simulink model "ct_finite_horizon"  (Simulink 8.7)
settings: Solver=ode45  StartTime=0.0  StopTime=5  MaxStep=1e-3  RelTol=1e-3
values from neighbouring files (symbols this model uses):
  p12 = fliplr(p12_acc)    [LUT_hint.m]    (also in Riccati_sol2.m)
  p22 = fliplr(p22_acc)    [LUT_hint.m]    (also in Riccati_sol2.m)
  Q = [2 1; 1 4]    [Riccati_sol2.m]    (also in file_for_LQR_EX.m = [100 0 ; 0 0]; inf_horiz.m = [10 0; 0 2000])
  R = 1/2    (= 0.5)    [Riccati_sol2.m]    (also in file_for_LQR_EX.m = 10; inf_horiz.m = 1)
  tt = fliplr(t_acc)    [LUT_hint.m]    (also in Riccati_sol2.m)
  Z = [p11_old p12_old; p12_old, p22_old]    [Riccati_sol2.m]
settings Model: Creator=Thomas Chmielewski  LastModifiedBy=DR_C
settings DataIOCC: SignalLoggingSaveFormat=ModelDataLogs  SignalLoggingName=sigsOut
settings OptimizationCC: ExpressionDepthLimit=2147483647  InitFltsAndDblsToZero=on
settings DebuggingCC: SaveWithParameterizedLinksMsg=none  SignalResolutionControl=TryResolveAllWithWarning  MultiTaskDSMMsg=warning  MultiTaskCondExecSysMsg=none  FcnCallInpInsideContextMsg=UseLocalSettings  StateNameClashWarn=warning
settings HardwareCC: TargetUnknown=on
settings GRTTargetCC: TargetFcnLib=ansi_tfl_tmw.mat  ModelReferenceCompliant=off  CombineOutputUpdateFcns=off  MatFileLogging=off  GRTInterface=on

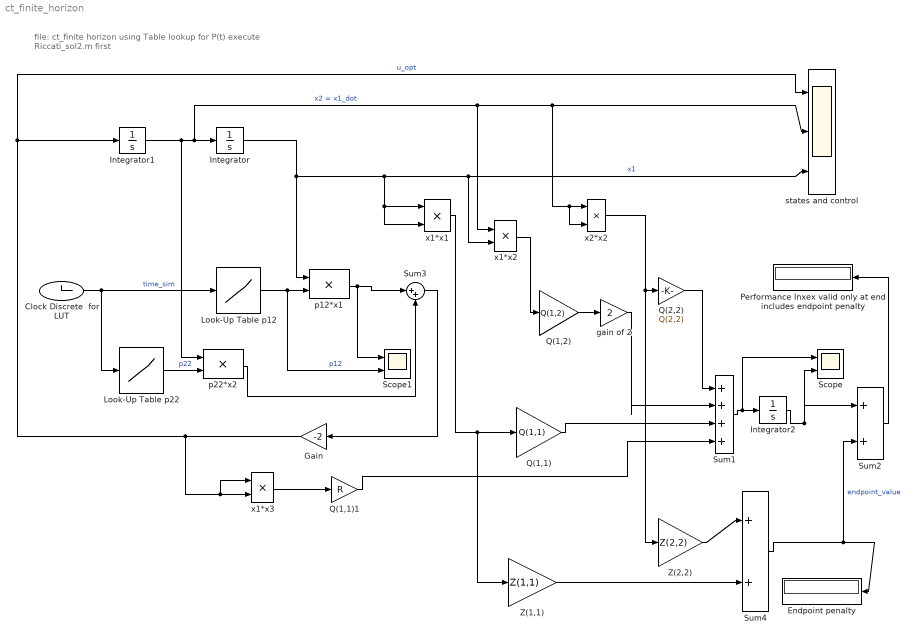
== system ct_finite_horizon ==
  note: file:  ct_finite horizon
      | using Table lookup for P(t) execute Riccati_sol2.m first
  Clock Discrete  for LUT : Clock
  Endpoint penalty : Display
  Gain : Gain  Gain=-2  SaturateOnIntegerOverflow=on  OutDataTypeStr=Inherit: Same as input  ParamDataTypeStr=Inherit: Same as input
  Integrator : Integrator  InitialCondition=10
  Integrator1 : Integrator  InitialCondition=10
  Integrator2 : Integrator
  Look-Up Table p12 : Lookup  InputValues=tt  Table=p12  SaturateOnIntegerOverflow=on
  Look-Up Table p22 : Lookup  InputValues=tt  Table=p22  SaturateOnIntegerOverflow=on
  "Performance Inxex valid only at end includes endpoint penalty " : Display
  Q(1,1) : Gain  Gain=Q(1,1)  SaturateOnIntegerOverflow=on  OutDataTypeStr=Inherit: Same as input  ParamDataTypeStr=Inherit: Same as input
  Q(1,1)1 : Gain  Gain=R  SaturateOnIntegerOverflow=on  OutDataTypeStr=Inherit: Same as input  ParamDataTypeStr=Inherit: Same as input
  Q(1,2) : Gain  Gain=Q(1,2)  SaturateOnIntegerOverflow=on  OutDataTypeStr=Inherit: Same as input  ParamDataTypeStr=Inherit: Same as input
  Q(2,2) : Gain  Gain=Q(2,2)  SaturateOnIntegerOverflow=on  OutDataTypeStr=Inherit: Same as input  ParamDataTypeStr=Inherit: Same as input
  Scope : Scope  NumInputPorts=2
  Scope1 : Scope  NumInputPorts=2
  Sum1 : Sum  Inputs=|++++  SaturateOnIntegerOverflow=on
  Sum2 : Sum  Inputs=|++  SaturateOnIntegerOverflow=on
  Sum3 : Sum  Inputs=|++  SaturateOnIntegerOverflow=on
  Sum4 : Sum  Inputs=|++  SaturateOnIntegerOverflow=on
  Z(1,1) : Gain  Gain=Z(1,1)  SaturateOnIntegerOverflow=on  OutDataTypeStr=Inherit: Same as input  ParamDataTypeStr=Inherit: Same as input
  Z(2,2) : Gain  Gain=Z(2,2)  SaturateOnIntegerOverflow=on  OutDataTypeStr=Inherit: Same as input  ParamDataTypeStr=Inherit: Same as input
  gain of 2 : Gain  Gain=2  SaturateOnIntegerOverflow=on  OutDataTypeStr=Inherit: Same as input  ParamDataTypeStr=Inherit: Same as input
  p12*x1 : Product  SaturateOnIntegerOverflow=on  OutDataTypeStr=Inherit: Same as first input
  p22*x2 : Product  SaturateOnIntegerOverflow=on  OutDataTypeStr=Inherit: Same as first input
  states and control : Scope  NumInputPorts=3
  x1*x1 : Product  SaturateOnIntegerOverflow=on  OutDataTypeStr=Inherit: Same as first input
  x1*x2 : Product  SaturateOnIntegerOverflow=on  OutDataTypeStr=Inherit: Same as first input
  x1*x3 : Product  SaturateOnIntegerOverflow=on  OutDataTypeStr=Inherit: Same as first input
  x2*x2 : Product  SaturateOnIntegerOverflow=on  OutDataTypeStr=Inherit: Same as first input
  wires:
  Integrator1/1 -> p22*x2/1, Integrator/1, x1*x2/1, states and control/2, x2*x2/2, x2*x2/1  "x2 = x1_dot"
  Integrator/1 -> p12*x1/1, states and control/3, x1*x2/2, x1*x1/2, x1*x1/1  "x1"
  Look-Up Table p12/1 -> p12*x1/2, Scope1/2  "p12"
  Look-Up Table p22/1 -> p22*x2/2  "p22"
  p12*x1/1 -> Sum3/1, Scope1/1
  p22*x2/1 -> Sum3/2
  Sum3/1 -> Gain/1
  Gain/1 -> Integrator1/1, states and control/1, x1*x3/2, x1*x3/1  "u_opt"
  Clock Discrete  for LUT/1 -> Look-Up Table p12/1, Look-Up Table p22/1  "time_sim"
  Sum4/1 -> Sum2/2, Endpoint penalty/1  "endpoint_value"
  Q(1,1)/1 -> Sum1/3
  x1*x1/1 -> Q(1,1)/1, Z(1,1)/1
  x1*x2/1 -> Q(1,2)/1
  Q(1,2)/1 -> gain of 2/1
  x2*x2/1 -> Q(2,2)/1, Z(2,2)/1
  Q(2,2)/1 -> Sum1/1
  Sum1/1 -> Integrator2/1, Scope/1
  Integrator2/1 -> Sum2/1, Scope/2
  Sum2/1 -> "Performance Inxex valid only at end includes endpoint penalty "/1
  Z(1,1)/1 -> Sum4/2
  Z(2,2)/1 -> Sum4/1
  x1*x3/1 -> Q(1,1)1/1
  Q(1,1)1/1 -> Sum1/4
  gain of 2/1 -> Sum1/2
